simulink model "pisSIMULINK"  (R2025b)
settings: Solver=VariableStepAuto  StartTime=0.0  StopTime=5  RelTol=1e-3
settings Model: Creator=JunioR  LastModifiedBy=JunioR

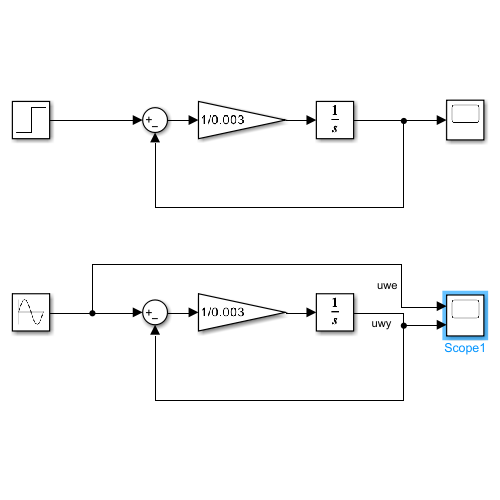
[thumbnail: Simulink's stored preview of the top-level diagram]
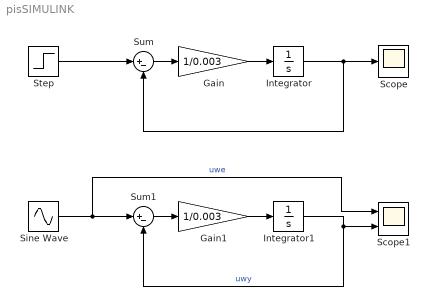
== system pisSIMULINK ==
  Gain : Gain  Gain=1/0.003
  Gain1 : Gain  Gain=1/0.003
  Integrator : Integrator
  Integrator1 : Integrator
  Scope : Scope
      settings: ActiveDisplayYMinimum=-0.1249878477035469  ActiveDisplayYMaximum=1.1248906293319223
  Scope1 : Scope  NumInputPorts=2
      settings: ActiveDisplayYMinimum=-4.1692864699369991  ActiveDisplayYMaximum=5.9088678397692531
  Sine Wave : Sin  Amplitude=50  Frequency=2*pi*1  SampleTime=0
  Step : Step  SampleTime=0
  Sum : Sum  Inputs=|+-
  Sum1 : Sum  Inputs=|+-
  wires:
  Step/1 -> Sum/1
  Sum/1 -> Gain/1
  Gain/1 -> Integrator/1
  Integrator/1 -> Sum/2, Scope/1
  Sum1/1 -> Gain1/1
  Gain1/1 -> Integrator1/1
  Sine Wave/1 -> Scope1/1, Sum1/1  "uwe"
  Integrator1/1 -> Sum1/2, Scope1/2  "uwy"
